simulink model "sst_spdab_npc_inv"  (R2025b)
settings: Solver=ode23tb  StartTime=0.0  StopTime=simlength  FixedStep=tc  MaxStep=tc
values from neighbouring files (symbols this model uses):
  Adrso = eye(2) + Arso*ts_inv    [init_model.m]
  Aresd_max = eye(2) + Ares_max*ts_afe    [init_model.m]
  Aresd_min = eye(2) + Ares_min*ts_afe    [init_model.m]
  Aresd_nom = eye(2) + Ares_nom*ts_afe    [init_model.m]
  Bresd = Bres*ts_afe    [init_model.m]
  CFi_dc2 = 900e-6*4    (= 0.0036)    [init_model.m]
  Cresd = Cres    [init_model.m]
  Crso = [1 0]    [init_model.m]
  delta = 0.025    [init_model.m]
  freq = 50    [init_model.m]
  Iac_FS = I_phase_normalization_factor    [init_model.m]
  Idc_FS = max(Idab1_dc_nom,Idab2_dc_nom) * margin_factor    [init_model.m]
  iph_grid_pu_ref = 3.75    [init_model.m]
  ki_afe = 18    [init_model.m]
  ki_pll = 3140    [init_model.m]
  ki_rpi = 18    [init_model.m]
  kp_afe = 0.25    [init_model.m]
  kp_pll = 314    [init_model.m]
  kp_rpi = 0.25    [init_model.m]
  Ldrso = acker(Adrso',Crso',polesdrso)'    [init_model.m]
  LFu1_AFE = 0.33e-3    (= 0.00033)    [init_model.m]
  n_modules = 2    [init_model.m]
  RLFu1_AFE = 157*0.05*LFu1_AFE    (= 0.0025905)    [init_model.m]
  tc = ts_dab/100    (= 1e-06)    [init_model.m]
  ts_afe = 1/fPWM_AFE    (= 0.0002)    [init_model.m]
  ts_inv = 1/fPWM_INV    (= 0.0002)    [init_model.m]
  Vac_FS = V_phase_normalization_factor    [init_model.m]
  Vdab2_dc_nom = 1500    [init_model.m]
  Vdc_FS = max(Vdab1_dc_nom,Vdab2_dc_nom) * margin_factor    [init_model.m]
undefined symbols (not defined in the file or in its folder): Ld2_trafo, omega_grid_nom, V_phase_normalization_factor
libraries: fl_lib x68, nesl_utility x40, pi_ctrl x4, discrete_time_low_pass_filter x4, dab_single_phase_pwm_modulator x2, full_bridge_mosfet_based_with_thermal_model x2, full_bridge_mosfet_based_with_thermal_model_zvs x2, single_phase_transformer x2, full_bridge_ideal_switch x2, dclink_for_three_levels x2, full_bridge_three_level_npc_ideal_switch_based_model x2, single_phase_three_levels_PWM_modulator x2
(part 3 of 4)

== system sst_spdab_npc_inv/dab_modB/dc//dc with galvanic isolation/full-bridge 1 ==
  gate_commands : Inport
  full-bridge ideal switch based : full_bridge_ideal_switch/full-bridge ideal switch based  Rds_on=Rds_on  Vdon_diode=Vdon_diode  Rdon_diode=Rdon_diode  Csnubber=Csnubber  Rsnubber=Rsnubber  Vth=7.5
  uac_1(+) : PMIOPort  Side=Left
  uac_1(-) : PMIOPort  Port=2  Side=Left
  Udc(+) : PMIOPort  Port=3  Side=Right
  Udc(-) : PMIOPort  Port=4  Side=Right
  wires:
  gate_commands/1 -> full-bridge ideal switch based/1
  connections:
  full-bridge ideal switch based/RConn1 -- uac_1(+)/RConn1
  full-bridge ideal switch based/RConn2 -- uac_1(-)/RConn1
  full-bridge ideal switch based/LConn2 -- Udc(-)/RConn1
  full-bridge ideal switch based/LConn1 -- Udc(+)/RConn1

== system sst_spdab_npc_inv/dab_modB/dc//dc with galvanic isolation/full-bridge 2 ==
  gate_commands : Inport
  CFi_dc2 : fl_lib/Electrical/Electrical Elements/Capacitor  c=CFi_dc2 F  r=RCFi_dc2_internal Ohm  g=0 1/Ohm  i_specify=off  i_priority=None  i=0 A  i_nominal_specify=off  i_nominal_value=1  i_nominal_unit=A  v_specify=off  v_priority=None  v=0 V  v_nominal_specify=off  v_nominal_value=1  v_nominal_unit=V  vc_specify=off  vc_priority=High  vc=0 V  vc_nominal_specify=off  vc_nominal_value=1  vc_nominal_unit=V
  Current Sensor2 : fl_lib/Electrical/Electrical Sensors/Current Sensor
  PS-Simulink Converter6 : nesl_utility/PS-Simulink Converter  PhysicalDomain=network_engine_domain  SubClassName=ps_output  LeftPortType=input  RightPortType=output  PseudoPeriodic=off  Frequencies=[]  VectorFormat=1-D array  Unit=A  AffineConversion=on
  full-bridge ideal switch based : full_bridge_ideal_switch/full-bridge ideal switch based  Rds_on=Rds_on  Vdon_diode=Vdon_diode  Rdon_diode=Rdon_diode  Csnubber=Csnubber  Rsnubber=Rsnubber  Vth=7.5
  uac_1(+) : PMIOPort  Side=Left
  uac_1(-) : PMIOPort  Port=2  Side=Left
  udc(+) : PMIOPort  Port=3  Side=Right
  udc(-) : PMIOPort  Port=4  Side=Right
  tag scope: CFi_dc2_current_modB=global
  wires:
  gate_commands/1 -> full-bridge ideal switch based/1
  PS-Simulink Converter6/1 -> [CFi_dc2_current_modB]  "CFi_dc2_current_modA"
  connections:
  CFi_dc2/LConn1 -- full-bridge ideal switch based/LConn1 -- udc(+)/RConn1
  Current Sensor2/RConn2 -- full-bridge ideal switch based/LConn2 -- udc(-)/RConn1
  PS-Simulink Converter6/LConn1 -- Current Sensor2/RConn1
  CFi_dc2/RConn1 -- Current Sensor2/LConn1
  uac_1(+)/RConn1 -- full-bridge ideal switch based/RConn1
  uac_1(-)/RConn1 -- full-bridge ideal switch based/RConn2

== system sst_spdab_npc_inv/dab_modB/dc//dc with galvanic isolation/scopes ==
  dab TR i2/i1 modB : Scope  NumInputPorts=2
      settings: SampleTime=tc  ActiveDisplayYMinimum=-993.52882611598045  ActiveDisplayYMaximum=1064.2487944856234  DataLoggingVariableName=ScopeData13
  dab TR u2/u1 modB : Scope  NumInputPorts=2
      settings: SampleTime=tc  ActiveDisplayYMinimum=-893.62031856834165  ActiveDisplayYMaximum=653.92363611228757  DataLoggingVariableName=ScopeData4
  dab current output/input modB : Scope  NumInputPorts=2
      settings: SampleTime=tc  ActiveDisplayYMinimum=-7335.7913745283768  ActiveDisplayYMaximum=23819.434208451414  DataLoggingVariableName=ScopeData8
  dab outputs modB : Scope  NumInputPorts=2
      settings: SampleTime=tc  ActiveDisplayYMinimum=-7444.4982322029246  ActiveDisplayYMaximum=21111.562445449617  DataLoggingVariableName=ScopeData6
  dab voltage input/output modB : Scope  NumInputPorts=2
      settings: SampleTime=tc  ActiveDisplayYMinimum=818.889253650666  ActiveDisplayYMaximum=1528.4588304760332  DataLoggingVariableName=ScopeData10
  wires:
  [dab_voltage_input_modB] -> dab voltage input/output modB/1  "dab_voltage_input_modB"
  [dab_current_output_modB] -> dab current output/input modB/1  "dab_current_output_modB"
  [dab_voltage_output_modB] -> dab voltage input/output modB/2  "dab_voltage_output_modB"
  [dab_current_input_modB] -> dab current output/input modB/2  "dab_current_input_modB"
  [i2_dab_transformer_modB] -> dab TR i2/i1 modB/1  "i2_dab_transformer_modB"
  [i1_dab_transformer_modB] -> dab TR i2/i1 modB/2  "i1_dab_transformer_modB"
  [u2_dab_transformer_modB] -> dab TR u2/u1 modB/1  "u2_dab_transformer_modB"
  [u1_dab_transformer_modB] -> dab TR u2/u1 modB/2  "u1_dab_transformer_modB"
  [dab_voltage_output_modB] -> dab outputs modB/2  "dab_voltage_output_modB"
  [dab_current_output_modB] -> dab outputs modB/1  "dab_current_output_modB"

== system sst_spdab_npc_inv/dab_modB/dc//dc with galvanic isolation/single_phase_dab_transformer ==
  Capacitor : fl_lib/Electrical/Electrical Elements/Capacitor  c=Cs1 F  r=1e-6 Ohm  g=0 1/Ohm  i_specify=off  i_priority=None  i=0 A  i_nominal_specify=off  i_nominal_value=1  i_nominal_unit=A  v_specify=off  v_priority=None  v=0 V  v_nominal_specify=off  v_nominal_value=1  v_nominal_unit=V  vc_specify=off  vc_priority=High  vc=0 V  vc_nominal_specify=off  vc_nominal_value=1  vc_nominal_unit=V
  Capacitor1 : fl_lib/Electrical/Electrical Elements/Capacitor  c=Cs2 F  r=1e-6 Ohm  g=0 1/Ohm  i_specify=off  i_priority=None  i=0 A  i_nominal_specify=off  i_nominal_value=1  i_nominal_unit=A  v_specify=off  v_priority=None  v=0 V  v_nominal_specify=off  v_nominal_value=1  v_nominal_unit=V  vc_specify=off  vc_priority=High  vc=0 V  vc_nominal_specify=off  vc_nominal_value=1  vc_nominal_unit=V
  Current Sensor : fl_lib/Electrical/Electrical Sensors/Current Sensor
  Current Sensor1 : fl_lib/Electrical/Electrical Sensors/Current Sensor
  Voltage Sensor1 : fl_lib/Electrical/Electrical Sensors/Voltage Sensor
  Voltage Sensor3 : fl_lib/Electrical/Electrical Sensors/Voltage Sensor
  i1_dab_transformer : nesl_utility/PS-Simulink Converter  PhysicalDomain=network_engine_domain  SubClassName=ps_output  LeftPortType=input  RightPortType=output  PseudoPeriodic=off  Frequencies=[]  VectorFormat=1-D array  Unit=A  AffineConversion=off
  i2_dab_transformer : nesl_utility/PS-Simulink Converter  PhysicalDomain=network_engine_domain  SubClassName=ps_output  LeftPortType=input  RightPortType=output  PseudoPeriodic=off  Frequencies=[]  VectorFormat=1-D array  Unit=A  AffineConversion=off
  single_phase_transformer : single_phase_transformer/single_phase_transformer  lm_trafo=lm_trafo  m1=m1  m2=m2  rd1_trafo=rd1_trafo  rd2_trafo=rd2_trafo  ld1_trafo=ld1_trafo  ld2_trafo=ld2_trafo  rfe_trafo=rfe_trafo  length_core=0.5  mu0=1.256637e-6  mur=70
  single_phase_transformer - scope : Scope
      settings: ActiveDisplayYMinimum=-6.2561553469400835  ActiveDisplayYMaximum=5.3110658573136256  DataLoggingVariableName=ScopeData20
  u1_dab_transformer : nesl_utility/PS-Simulink Converter  PhysicalDomain=network_engine_domain  SubClassName=ps_output  LeftPortType=input  RightPortType=output  PseudoPeriodic=off  Frequencies=[]  VectorFormat=1-D array  Unit=V  AffineConversion=on
  u2_dab_transformer : nesl_utility/PS-Simulink Converter  PhysicalDomain=network_engine_domain  SubClassName=ps_output  LeftPortType=input  RightPortType=output  PseudoPeriodic=off  Frequencies=[]  VectorFormat=1-D array  Unit=V  AffineConversion=on
  u1(+) : PMIOPort  Side=Left
  u2(+) : PMIOPort  Port=2  Side=Right
  u1(-) : PMIOPort  Port=3  Side=Left
  u2(-) : PMIOPort  Port=4  Side=Right
  tag scope: i1_dab_transformer_modB=global, i2_dab_transformer_modB=global, u1_dab_transformer_modB=global, u2_dab_transformer_modB=global
  wires:
  i2_dab_transformer/1 -> [i2_dab_transformer_modB]
  u2_dab_transformer/1 -> [u2_dab_transformer_modB]
  u1_dab_transformer/1 -> [u1_dab_transformer_modB]
  i1_dab_transformer/1 -> [i1_dab_transformer_modB]
  single_phase_transformer/1 -> single_phase_transformer - scope/1
  connections:
  Current Sensor/RConn2 -- u2(+)/RConn1
  Voltage Sensor3/RConn2 -- single_phase_transformer/RConn2 -- u2(-)/RConn1
  Current Sensor/RConn1 -- i2_dab_transformer/LConn1
  Voltage Sensor3/RConn1 -- u2_dab_transformer/LConn1
  Voltage Sensor1/RConn2 -- single_phase_transformer/LConn2 -- u1(-)/RConn1
  Current Sensor1/LConn1 -- Voltage Sensor1/LConn1 -- u1(+)/RConn1
  Voltage Sensor1/RConn1 -- u1_dab_transformer/LConn1
  Current Sensor1/RConn1 -- i1_dab_transformer/LConn1
  Voltage Sensor3/LConn1 -- Capacitor1/RConn1 -- Current Sensor/LConn1
  Capacitor/LConn1 -- Current Sensor1/RConn2
  single_phase_transformer/LConn1 -- Capacitor/RConn1
  single_phase_transformer/RConn1 -- Capacitor1/LConn1

== system sst_spdab_npc_inv/inverter_modA/single phase inverter control1/acquisition_and_scaling_current ==
  in : Inport
  1/Ti5 : Gain  Gain=1/Iac_FS  SaturateOnIntegerOverflow=on  OutDataTypeStr=Inherit: Same as input  ParamDataTypeStr=Inherit: Same as input
  out : Outport
  wires:
  in/1 -> 1/Ti5/1
  1/Ti5/1 -> out/1

== system sst_spdab_npc_inv/inverter_modA/single phase inverter control1/acquisition_and_scaling_dc_voltage ==
  in : Inport
  1/Ti3 : Gain  Gain=1/Vdc_FS  SaturateOnIntegerOverflow=on  OutDataTypeStr=Inherit: Same as input  ParamDataTypeStr=Inherit: Same as input
  out : Outport
  wires:
  in/1 -> 1/Ti3/1
  1/Ti3/1 -> out/1

== system sst_spdab_npc_inv/inverter_modA/single phase inverter control1/acquisition_and_scaling_voltage ==
  in : Inport
  1/Ti5 : Gain  Gain=1/Vac_FS  SaturateOnIntegerOverflow=on  OutDataTypeStr=Inherit: Same as input  ParamDataTypeStr=Inherit: Same as input
  out : Outport
  wires:
  in/1 -> 1/Ti5/1
  1/Ti5/1 -> out/1

== system sst_spdab_npc_inv/inverter_modA/single phase inverter control1/acquisition_and_scaling_voltage1 ==
  in : Inport
  1/Ti1 : Gain  Gain=1/Vac_FS  SaturateOnIntegerOverflow=on  OutDataTypeStr=Inherit: Same as input  ParamDataTypeStr=Inherit: Same as input
  1/Ti2 : Gain  Gain=1/n_modules  SaturateOnIntegerOverflow=on  OutDataTypeStr=Inherit: Same as input  ParamDataTypeStr=Inherit: Same as input
  out : Outport
  wires:
  in/1 -> 1/Ti2/1
  1/Ti1/1 -> out/1
  1/Ti2/1 -> 1/Ti1/1

== system sst_spdab_npc_inv/inverter_modA/single phase inverter control1/inverter_current_output_pu_reference ==
  Gain : Gain  Gain=-1
  Rate Limiter : RateLimiter  RisingSlewLimit=50  FallingSlewLimit=-50  SampleTimeMode=inherited
  Sum : Sum  Inputs=|++
  i_out_inverter_reference_step1 : Step  Time=0.05  After=iph_grid_pu_ref  SampleTime=0
  i_out_inverter_reference_step2 : Step  Commented=on  Time=0.25  After=-iph_grid_pu_ref  SampleTime=0
  inverter_current_output_pu_reference : Outport
  wires:
  Rate Limiter/1 -> Gain/1
  Sum/1 -> Rate Limiter/1
  i_out_inverter_reference_step1/1 -> Sum/1
  i_out_inverter_reference_step2/1 -> Sum/2
  Gain/1 -> inverter_current_output_pu_reference/1

== system sst_spdab_npc_inv/inverter_modA/single phase inverter control1/pwm modulator ==
  vout : Inport
  Constant : Constant  Value=0
  single_phase_three_levels_PWM_generator_with_global_TRGO : single_phase_three_levels_PWM_modulator/single_phase_three_levels_PWM_generator_with_global_TRGO  f=fPWM_INV  m_up=1  m_low=-1  dead_time=dead_time_INV  pos_cmd_gate=15  neg_cmd_gate=-10  polarity=1  tc=tc  double_sampling=TRGO_double_update
  gate_cmds : Outport
  tag scope: TRGO_INV_1=global
  wires:
  vout/1 -> single_phase_three_levels_PWM_generator_with_global_TRGO/3
  [time_afe_module_1] -> single_phase_three_levels_PWM_generator_with_global_TRGO/1
  Constant/1 -> single_phase_three_levels_PWM_generator_with_global_TRGO/2
  single_phase_three_levels_PWM_generator_with_global_TRGO/2 -> gate_cmds/1
  single_phase_three_levels_PWM_generator_with_global_TRGO/1 -> [TRGO_INV_1]

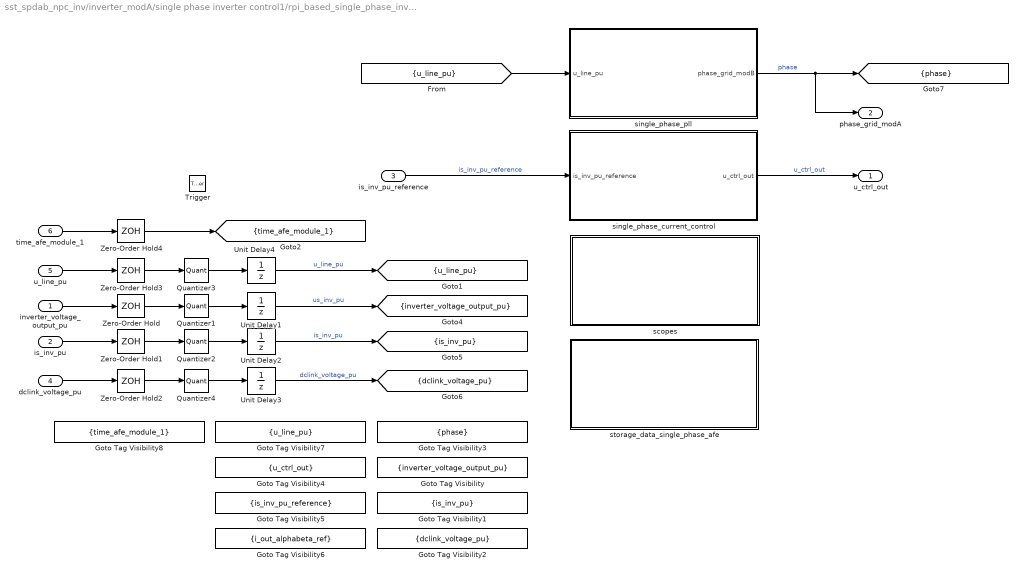
== system sst_spdab_npc_inv/inverter_modA/single phase inverter control1/rpi_based_single_phase_inverter_ctrl ==
  inverter_voltage_output_pu : Inport
  is_inv_pu : Inport  Port=2
  is_inv_pu_reference : Inport  Port=3
  dclink_voltage_pu : Inport  Port=4
  u_line_pu : Inport  Port=5
  time_afe_module_1 : Inport  Port=6
  Trigger : TriggerPort  VariantControl=(inherit)  PortDimensions=1
  Goto Tag Visibility : GotoTagVisibility  GotoTag=inverter_voltage_output_pu
  Goto Tag Visibility1 : GotoTagVisibility  GotoTag=is_inv_pu
  Goto Tag Visibility2 : GotoTagVisibility  GotoTag=dclink_voltage_pu
  Goto Tag Visibility3 : GotoTagVisibility  GotoTag=phase
  Goto Tag Visibility4 : GotoTagVisibility  GotoTag=u_ctrl_out
  Goto Tag Visibility5 : GotoTagVisibility  GotoTag=is_inv_pu_reference
  Goto Tag Visibility6 : GotoTagVisibility  GotoTag=i_out_alphabeta_ref
  Goto Tag Visibility7 : GotoTagVisibility  GotoTag=u_line_pu
  Goto Tag Visibility8 : GotoTagVisibility  GotoTag=time_afe_module_1
  Quantizer{1..4} (4 alike) : Quantizer  QuantizationInterval=adc12_quantization
  Unit Delay{1..4} (4 alike) : UnitDelay  SampleTime=-1  HasFrameUpgradeWarning=on
  Zero-Order Hold{,1..4} (5 alike) : ZeroOrderHold  SampleTime=-1
  scopes : Subsystem
  single_phase_current_control : Subsystem
  single_phase_pll : Subsystem
  storage_data_single_phase_afe : Subsystem
  u_ctrl_out : Outport
  phase_grid_modA : Outport  Port=2
  tag scope: dclink_voltage_pu=scoped, inverter_voltage_output_pu=scoped, is_inv_pu=scoped, phase=scoped, time_afe_module_1=scoped, u_line_pu=scoped
  wires:
  inverter_voltage_output_pu/1 -> Zero-Order Hold/1
  is_inv_pu/1 -> Zero-Order Hold1/1
  dclink_voltage_pu/1 -> Zero-Order Hold2/1
  Unit Delay1/1 -> [inverter_voltage_output_pu]  "us_inv_pu"
  Unit Delay2/1 -> [is_inv_pu]  "is_inv_pu"
  Unit Delay3/1 -> [dclink_voltage_pu]  "dclink_voltage_pu"
  is_inv_pu_reference/1 -> single_phase_current_control/1(is_inv_pu_reference)  "is_inv_pu_reference"
  single_phase_current_control/1(u_ctrl_out) -> u_ctrl_out/1  "u_ctrl_out"
  u_line_pu/1 -> Zero-Order Hold3/1
  Quantizer1/1 -> Unit Delay1/1
  Quantizer2/1 -> Unit Delay2/1
  Quantizer4/1 -> Unit Delay3/1
  Quantizer3/1 -> Unit Delay4/1
  single_phase_pll/1(phase_grid_modB) -> phase_grid_modA/1, [phase]  "phase"
  Zero-Order Hold/1 -> Quantizer1/1
  Zero-Order Hold1/1 -> Quantizer2/1
  Zero-Order Hold2/1 -> Quantizer4/1
  Unit Delay4/1 -> [u_line_pu]  "u_line_pu"
  [u_line_pu] -> single_phase_pll/1(u_line_pu)
  Zero-Order Hold3/1 -> Quantizer3/1
  time_afe_module_1/1 -> Zero-Order Hold4/1
  Zero-Order Hold4/1 -> [time_afe_module_1]

== system sst_spdab_npc_inv/inverter_modB/single phase inverter control1/acquisition_and_scaling_current ==
  in : Inport
  1/Ti5 : Gain  Gain=1/Iac_FS  SaturateOnIntegerOverflow=on  OutDataTypeStr=Inherit: Same as input  ParamDataTypeStr=Inherit: Same as input
  out : Outport
  wires:
  in/1 -> 1/Ti5/1
  1/Ti5/1 -> out/1

== system sst_spdab_npc_inv/inverter_modB/single phase inverter control1/acquisition_and_scaling_dc_voltage ==
  in : Inport
  1/Ti3 : Gain  Gain=1/Vdc_FS  SaturateOnIntegerOverflow=on  OutDataTypeStr=Inherit: Same as input  ParamDataTypeStr=Inherit: Same as input
  out : Outport
  wires:
  in/1 -> 1/Ti3/1
  1/Ti3/1 -> out/1

== system sst_spdab_npc_inv/inverter_modB/single phase inverter control1/acquisition_and_scaling_voltage ==
  in : Inport
  1/Ti5 : Gain  Gain=1/Vac_FS  SaturateOnIntegerOverflow=on  OutDataTypeStr=Inherit: Same as input  ParamDataTypeStr=Inherit: Same as input
  out : Outport
  wires:
  in/1 -> 1/Ti5/1
  1/Ti5/1 -> out/1

== system sst_spdab_npc_inv/inverter_modB/single phase inverter control1/acquisition_and_scaling_voltage1 ==
  in : Inport
  1/Ti1 : Gain  Gain=1/Vac_FS  SaturateOnIntegerOverflow=on  OutDataTypeStr=Inherit: Same as input  ParamDataTypeStr=Inherit: Same as input
  1/Ti2 : Gain  Gain=1/n_modules  SaturateOnIntegerOverflow=on  OutDataTypeStr=Inherit: Same as input  ParamDataTypeStr=Inherit: Same as input
  out : Outport
  wires:
  in/1 -> 1/Ti2/1
  1/Ti1/1 -> out/1
  1/Ti2/1 -> 1/Ti1/1

== system sst_spdab_npc_inv/inverter_modB/single phase inverter control1/inverter_current_output_pu_reference ==
  Gain : Gain
  Rate Limiter : RateLimiter  RisingSlewLimit=50  FallingSlewLimit=-50  SampleTimeMode=inherited
  Sum : Sum  Inputs=|++
  i_out_inverter_reference_step1 : Step  Time=0.05  After=iph_grid_pu_ref  SampleTime=0
  i_out_inverter_reference_step2 : Step  Commented=on  Time=0.25  After=-iph_grid_pu_ref  SampleTime=0
  inverter_current_output_pu_reference : Outport
  wires:
  Rate Limiter/1 -> Gain/1
  Sum/1 -> Rate Limiter/1
  i_out_inverter_reference_step1/1 -> Sum/1
  i_out_inverter_reference_step2/1 -> Sum/2
  Gain/1 -> inverter_current_output_pu_reference/1

== system sst_spdab_npc_inv/inverter_modB/single phase inverter control1/pwm modulator ==
  vout : Inport
  Constant : Constant  Value=0
  single_phase_three_levels_PWM_generator_with_global_TRGO : single_phase_three_levels_PWM_modulator/single_phase_three_levels_PWM_generator_with_global_TRGO  f=fPWM_INV  m_up=1  m_low=-1  dead_time=dead_time_INV  pos_cmd_gate=15  neg_cmd_gate=-10  polarity=1  tc=tc  double_sampling=TRGO_double_update
  gate_cmds : Outport
  tag scope: TRGO_INV_2=global
  wires:
  vout/1 -> single_phase_three_levels_PWM_generator_with_global_TRGO/3
  Constant/1 -> single_phase_three_levels_PWM_generator_with_global_TRGO/2
  single_phase_three_levels_PWM_generator_with_global_TRGO/2 -> gate_cmds/1
  single_phase_three_levels_PWM_generator_with_global_TRGO/1 -> [TRGO_INV_2]
  [time_afe_module_2] -> single_phase_three_levels_PWM_generator_with_global_TRGO/1

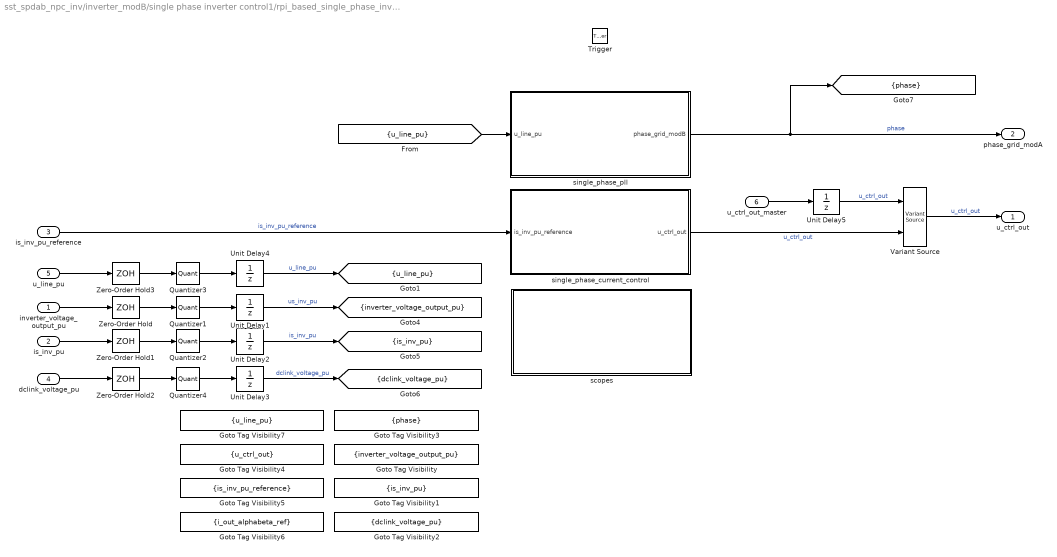
== system sst_spdab_npc_inv/inverter_modB/single phase inverter control1/rpi_based_single_phase_inverter_ctrl ==
  inverter_voltage_output_pu : Inport
  is_inv_pu : Inport  Port=2
  is_inv_pu_reference : Inport  Port=3
  dclink_voltage_pu : Inport  Port=4
  u_line_pu : Inport  Port=5
  u_ctrl_out_master : Inport  Port=6
  Trigger : TriggerPort  VariantControl=(inherit)  PortDimensions=1
  Goto Tag Visibility : GotoTagVisibility  GotoTag=inverter_voltage_output_pu
  Goto Tag Visibility1 : GotoTagVisibility  GotoTag=is_inv_pu
  Goto Tag Visibility2 : GotoTagVisibility  GotoTag=dclink_voltage_pu
  Goto Tag Visibility3 : GotoTagVisibility  GotoTag=phase
  Goto Tag Visibility4 : GotoTagVisibility  GotoTag=u_ctrl_out
  Goto Tag Visibility5 : GotoTagVisibility  GotoTag=is_inv_pu_reference
  Goto Tag Visibility6 : GotoTagVisibility  GotoTag=i_out_alphabeta_ref
  Goto Tag Visibility7 : GotoTagVisibility  GotoTag=u_line_pu
  Quantizer{1..4} (4 alike) : Quantizer  QuantizationInterval=adc12_quantization
  Unit Delay{1..5} (5 alike) : UnitDelay  SampleTime=-1  HasFrameUpgradeWarning=on
  Variant Source : VariantSource  VariantControls={true, false}
  Zero-Order Hold{,1..3} (4 alike) : ZeroOrderHold  SampleTime=-1
  scopes : Subsystem
  single_phase_current_control : Subsystem
  single_phase_pll : Subsystem
  u_ctrl_out : Outport
  phase_grid_modA : Outport  Port=2
  tag scope: dclink_voltage_pu=scoped, inverter_voltage_output_pu=scoped, is_inv_pu=scoped, phase=scoped, u_line_pu=scoped
  wires:
  inverter_voltage_output_pu/1 -> Zero-Order Hold/1
  is_inv_pu/1 -> Zero-Order Hold1/1
  dclink_voltage_pu/1 -> Zero-Order Hold2/1
  Unit Delay1/1 -> [inverter_voltage_output_pu]  "us_inv_pu"
  Unit Delay2/1 -> [is_inv_pu]  "is_inv_pu"
  Unit Delay3/1 -> [dclink_voltage_pu]  "dclink_voltage_pu"
  is_inv_pu_reference/1 -> single_phase_current_control/1(is_inv_pu_reference)  "is_inv_pu_reference"
  u_line_pu/1 -> Zero-Order Hold3/1
  Quantizer1/1 -> Unit Delay1/1
  Quantizer2/1 -> Unit Delay2/1
  Quantizer4/1 -> Unit Delay3/1
  Quantizer3/1 -> Unit Delay4/1
  single_phase_pll/1(phase_grid_modB) -> [phase], phase_grid_modA/1  "phase"
  Zero-Order Hold/1 -> Quantizer1/1
  Zero-Order Hold1/1 -> Quantizer2/1
  Zero-Order Hold2/1 -> Quantizer4/1
  Unit Delay4/1 -> [u_line_pu]  "u_line_pu"
  [u_line_pu] -> single_phase_pll/1(u_line_pu)
  Zero-Order Hold3/1 -> Quantizer3/1
  u_ctrl_out_master/1 -> Unit Delay5/1
  Unit Delay5/1 -> Variant Source/1  "u_ctrl_out"
  Variant Source/1 -> u_ctrl_out/1  "u_ctrl_out"
  single_phase_current_control/1(u_ctrl_out) -> Variant Source/2  "u_ctrl_out"

== system sst_spdab_npc_inv/dab_modA/dab_ctrl/dab_voltage&current_controllers/input current controller ==
  i_in_dab_ref : Inport
  i_in_dab : Inport  Port=2
  Gain : Gain
  dab_current_control performance_modA : Scope  NumInputPorts=3
      settings: ActiveDisplayYMinimum=-1.3198512407012277  ActiveDisplayYMaximum=3.2550260581251234  DataLoggingVariableName=ScopeData12
  pi_ctrl : pi_ctrl/pi_ctrl  kp=kp_i_dab  ki=ki_i_dab  ts=ts_dab  lim_up=1  lim_down=-1
  i_ctrl_out : Outport
  wires:
  i_in_dab_ref/1 -> pi_ctrl/1, dab_current_control performance_modA/1, Gain/1  "i_in_dab_ref"
  i_in_dab/1 -> pi_ctrl/2, dab_current_control performance_modA/2  "i_in_dab"
  pi_ctrl/1 -> i_ctrl_out/1, dab_current_control performance_modA/3  "i_ctrl_out"
  Gain/1 -> pi_ctrl/3

== system sst_spdab_npc_inv/dab_modA/dab_ctrl/dab_voltage&current_controllers/output voltage controller ==
  u_out_dab_ref : Inport
  u_out_dab : Inport  Port=2
  dab_voltage_control performance_modA : Scope  NumInputPorts=3
      settings: ActiveDisplayYMinimum=-1.3198512407012277  ActiveDisplayYMaximum=3.2550260581251234  DataLoggingVariableName=ScopeData14
  pi_ctrl : pi_ctrl/pi_ctrl  kp=kp_v_dab  ki=ki_v_dab  ts=ts_dab  lim_up=4  lim_down=-4
  u_ctrl_out : Outport
  wires:
  u_out_dab/1 -> dab_voltage_control performance_modA/2, pi_ctrl/2  "u_out_dab"
  u_out_dab_ref/1 -> dab_voltage_control performance_modA/1, pi_ctrl/1  "u_out_dab_ref"
  pi_ctrl/1 -> dab_voltage_control performance_modA/3, u_ctrl_out/1  "u_ctrl_out"

== system sst_spdab_npc_inv/dab_modA/dab_ctrl/dab_voltage&current_controllers/scopes ==
  Bus Creator : BusCreator  Inputs=2
  Bus Creator1 : BusCreator  Inputs=2
  dab-tracking modA : Scope  NumInputPorts=2
      settings: ActiveDisplayYMinimum=-2.2033655574404327  ActiveDisplayYMaximum=2.9011172646804795  DataLoggingVariableName=ScopeData7
  u_ctrl_out_dab/i_ctrl_out_dab modA : Scope  NumInputPorts=2
      settings: ActiveDisplayYMinimum=-1.25  ActiveDisplayYMaximum=1.25
  wires:
  [dab_current_input_pu] -> Bus Creator1/2  "dab_current_input_pu"
  [dab_current_ctrl_output_pu] -> u_ctrl_out_dab/i_ctrl_out_dab modA/2  "i_ctrl_out_dab"
  [dab_voltage_output_pu] -> Bus Creator/2  "dab_voltage_output_pu"
  [dab_voltage_output_pu_reference] -> Bus Creator/1  "dab_current_input_pu_ref"
  Bus Creator1/1 -> dab-tracking modA/2
  Bus Creator/1 -> dab-tracking modA/1
  [dab_voltage_ctrl_output_pu] -> u_ctrl_out_dab/i_ctrl_out_dab modA/1  "u_ctrl_out_dab"
  [dab_voltage_ctrl_output_pu] -> Bus Creator1/1  "u_ctrl_out_dab"

== system sst_spdab_npc_inv/dab_modA/dab_ctrl/dab_voltage&current_controllers/storage_data_dab ==
  To Workspace1 : ToWorkspace  VariableName=time_ts_dab_sim  SampleTime=-1
      settings: MaxDataPoints=Ns_dab
  To Workspace2 : ToWorkspace  VariableName=dab_current_input_pu_ref_sim  SampleTime=-1
      settings: MaxDataPoints=Ns_dab
  To Workspace3 : ToWorkspace  VariableName=dab_voltage_output_pu_sim  SampleTime=-1
      settings: MaxDataPoints=Ns_dab
  To Workspace5 : ToWorkspace  VariableName=dab_current_input_pu_sim  SampleTime=-1
      settings: MaxDataPoints=Ns_dab
  To Workspace6 : ToWorkspace  VariableName=u_ctrl_out_dab_sim  SampleTime=-1
      settings: MaxDataPoints=Ns_dab
  To Workspace7 : ToWorkspace  VariableName=i_ctrl_out_dab_sim  SampleTime=-1
      settings: MaxDataPoints=Ns_dab
  wires:
  [dab_voltage_ctrl_output_pu] -> To Workspace6/1  "u_ctrl_out_dab"
  [dab_voltage_output_pu_reference] -> To Workspace2/1  "dab_current_input_pu_ref"
  [dab_voltage_output_pu] -> To Workspace3/1  "dab_voltage_output_pu"
  [dab_current_ctrl_output_pu] -> To Workspace7/1  "i_ctrl_out_dab"
  [dab_current_input_pu] -> To Workspace5/1  "dab_current_input_pu"
  [time_dab_module_1] -> To Workspace1/1

== system sst_spdab_npc_inv/dab_modB/dab_ctrl/dab_voltage&current_controllers/input current controller ==
  i_in_dab_ref : Inport
  i_in_dab : Inport  Port=2
  Gain : Gain
  dab_current_control performance_modB : Scope  NumInputPorts=3
      settings: ActiveDisplayYMinimum=-1.3198512407012277  ActiveDisplayYMaximum=3.2550260581251234  DataLoggingVariableName=ScopeData12
  pi_ctrl : pi_ctrl/pi_ctrl  kp=kp_i_dab  ki=ki_i_dab  ts=ts_dab  lim_up=1  lim_down=-1
  i_ctrl_out : Outport
  wires:
  i_in_dab_ref/1 -> pi_ctrl/1, dab_current_control performance_modB/1, Gain/1  "i_in_dab_ref"
  i_in_dab/1 -> pi_ctrl/2, dab_current_control performance_modB/2  "i_in_dab"
  pi_ctrl/1 -> i_ctrl_out/1, dab_current_control performance_modB/3  "i_ctrl_out"
  Gain/1 -> pi_ctrl/3

== system sst_spdab_npc_inv/dab_modB/dab_ctrl/dab_voltage&current_controllers/output voltage controller ==
  u_out_dab_ref : Inport
  u_out_dab : Inport  Port=2
  dab_voltage_control performance_modB : Scope  NumInputPorts=3
      settings: ActiveDisplayYMinimum=-0.72078430609168342  ActiveDisplayYMaximum=1.2253779437324093  DataLoggingVariableName=ScopeData14
  pi_ctrl : pi_ctrl/pi_ctrl  kp=kp_v_dab  ki=ki_v_dab  ts=ts_dab  lim_up=4  lim_down=-4
  u_ctrl_out : Outport
  wires:
  u_out_dab/1 -> dab_voltage_control performance_modB/2, pi_ctrl/2  "u_out_dab"
  u_out_dab_ref/1 -> dab_voltage_control performance_modB/1, pi_ctrl/1  "u_out_dab_ref"
  pi_ctrl/1 -> dab_voltage_control performance_modB/3, u_ctrl_out/1  "u_ctrl_out"

== system sst_spdab_npc_inv/dab_modB/dab_ctrl/dab_voltage&current_controllers/scopes ==
  Bus Creator : BusCreator  Inputs=2
  Bus Creator1 : BusCreator  Inputs=2
  dab-tracking modB : Scope  NumInputPorts=2
      settings: ActiveDisplayYMinimum=-2.2033655574404327  ActiveDisplayYMaximum=2.9011172646804795  DataLoggingVariableName=ScopeData7
  u_ctrl_out_dab/i_ctrl_out_dab modB : Scope  NumInputPorts=2
      settings: ActiveDisplayYMinimum=-1.25  ActiveDisplayYMaximum=1.25
  wires:
  [dab_current_input_pu] -> Bus Creator1/2  "dab_current_input_pu"
  [dab_current_ctrl_output_pu] -> u_ctrl_out_dab/i_ctrl_out_dab modB/2  "i_ctrl_out_dab"
  [dab_voltage_output_pu] -> Bus Creator/2  "dab_voltage_output_pu"
  [dab_voltage_output_pu_reference] -> Bus Creator/1  "dab_current_input_pu_ref"
  Bus Creator1/1 -> dab-tracking modB/2
  Bus Creator/1 -> dab-tracking modB/1
  [dab_voltage_ctrl_output_pu] -> u_ctrl_out_dab/i_ctrl_out_dab modB/1  "u_ctrl_out_dab"
  [dab_voltage_ctrl_output_pu] -> Bus Creator1/1  "u_ctrl_out_dab"

== system sst_spdab_npc_inv/inverter_modA/single phase inverter control1/rpi_based_single_phase_inverter_ctrl/scopes ==
  Bus Creator1 : BusCreator  Inputs=3
  Bus Creator2 : BusCreator  Inputs=2
  Bus Creator3 : BusCreator  Inputs=2
  Bus Creator4 : BusCreator  Inputs=2
  single phase inverter tracking current scope 1 : Scope  NumInputPorts=2
      settings: ActiveDisplayYMinimum=-3.13873291015625  ActiveDisplayYMaximum=3.12652587890625  DataLoggingVariableName=ScopeData12
  single phase inverter tracking current scope 2 : Scope  NumInputPorts=2
      settings: ActiveDisplayYMinimum=-9.9064807170854827  ActiveDisplayYMaximum=9.6151714521585063  DataLoggingVariableName=ScopeData2
  single phase inverter tracking current scope 3 : Scope  NumInputPorts=2
      settings: ActiveDisplayYMinimum=-9.9064807170854827  ActiveDisplayYMaximum=9.6151714521585063  DataLoggingVariableName=ScopeData21
  wires:
  Bus Creator1/1 -> single phase inverter tracking current scope 1/2  "is_tracking"
  [i_out_alphabeta_ref] -> Bus Creator1/2  "i_out_inverter_pu_ref"
  [is_inv_pu] -> Bus Creator1/3  "inverter_current_output_pu"
  [inverter_voltage_output_pu] -> Bus Creator2/1  "inverter_voltage_output_pu"
  Bus Creator2/1 -> single phase inverter tracking current scope 1/1  "load"
  [is_inv_pu_reference] -> Bus Creator1/1  "inverter_current_output_pu_reference"
  [is_inv_pu] -> Bus Creator2/2  "inverter_current_output_pu"
  [u_ctrl_out] -> Bus Creator3/1  "u_ctrl_out"
  [inverter_voltage_output_pu] -> Bus Creator3/2  "inverter_voltage_output_pu"
  Bus Creator3/1 -> single phase inverter tracking current scope 2/2  "u_load"
  [is_inv_pu] -> Bus Creator4/2  "inverter_current_output_pu"
  [i_out_alphabeta_ref] -> Bus Creator4/1  "i_out_alphabeta_ref"
  Bus Creator4/1 -> single phase inverter tracking current scope 2/1  "i_load"
  [phase] -> single phase inverter tracking current scope 3/1  "phase_pll"

== system sst_spdab_npc_inv/inverter_modA/single phase inverter control1/rpi_based_single_phase_inverter_ctrl/single_phase_current_control ==
  is_inv_pu_reference : Inport
  Variant Source : VariantSource  VariantControls={rpi_enable == 1, rpi_enable == 0}
  current_reference_generation : Subsystem
  dqpi_current_controller : Subsystem
  rpi_current_controller : Subsystem
  u_ctrl_out : Outport
  tag scope: i_out_alphabeta_ref=scoped, is_inv_pu_reference=scoped, u_ctrl_out=scoped
  wires:
  rpi_current_controller/1(u_ctrl_out) -> Variant Source/1  "u_ctrl_out"
  dqpi_current_controller/1(u_out) -> Variant Source/2  "u_ctrl_out"
  current_reference_generation/1(is_ref) -> rpi_current_controller/1(i_ref), [i_out_alphabeta_ref]  "i_out_inverter_pu_ref"
  Variant Source/1 -> u_ctrl_out/1, [u_ctrl_out]  "u_ctrl_out"
  [phase] -> current_reference_generation/2(phase)
  is_inv_pu_reference/1 -> current_reference_generation/1(mag_ref), [is_inv_pu_reference]
  current_reference_generation/2(idc_ref) -> dqpi_current_controller/1(i_ref)

== system sst_spdab_npc_inv/inverter_modA/single phase inverter control1/rpi_based_single_phase_inverter_ctrl/single_phase_pll ==
  u_line_pu : Inport
  Constant : Constant  Value=2*pi*freq
  Constant2 : Constant  Value=0
  Sum : Sum  Inputs=|++
  Sum1 : Sum  Inputs=|++
  Terminator1 : Terminator
  Terminator2 : Terminator
  Terminator3 : Terminator
  Unit Delay1 : UnitDelay  SampleTime=-1  HasFrameUpgradeWarning=on
  alphabeta2xieta : MATLAB Function  TreatAsAtomicUnit=on
  double_integrator_observer : Subsystem
  freq_pll : Gain  Gain=1/2/pi
  omega_int_ts : Gain  Gain=ts_inv
  pi-ctrl : Subsystem  mask{kp=kp_pll, ki=ki_pll, ts=ts_afe, sat_pos=inf, sat_neg=-inf}
  theta_pll_hat : Gain
  ualpha_pll : Gain
  ubeta_pll : Gain
  ueta_pll : Gain  Gain=-1
  ueta_pll_flt : discrete_time_low_pass_filter/discrete-time-low-pass-filter  tau=tau_f  ts=ts_afe
  uxi_pll : Gain
  uxi_pll_flt : discrete_time_low_pass_filter/discrete-time-low-pass-filter  tau=tau_f  ts=ts_afe
  xieta2alphabeta : MATLAB Function  TreatAsAtomicUnit=on
  phase_grid_modB : Outport
  wires:
  Sum/1 -> Unit Delay1/1
  alphabeta2xieta/1(xi) -> uxi_pll_flt/1, uxi_pll/1
  xieta2alphabeta/2(beta) -> ubeta_pll/1
  alphabeta2xieta/2(eta) -> ueta_pll_flt/1, ueta_pll/1
  omega_int_ts/1 -> Sum/1
  double_integrator_observer/1(theta_hat) -> theta_pll_hat/1  "theta_hat"
  u_line_pu/1 -> alphabeta2xieta/1(alpha)
  freq_pll/1 -> Terminator1/1  "freq_pll"
  ueta_pll_flt/1 -> xieta2alphabeta/2(eta)
  uxi_pll_flt/1 -> xieta2alphabeta/1(xi)
  ueta_pll/1 -> pi-ctrl/1(x)
  Sum1/1 -> freq_pll/1, omega_int_ts/1  "freq_pll"
  Constant2/1 -> pi-ctrl/2(xref)
  uxi_pll/1 -> Terminator2/1
  ubeta_pll/1 -> alphabeta2xieta/2(beta)
  xieta2alphabeta/1(alpha) -> ualpha_pll/1
  ualpha_pll/1 -> Terminator3/1
  pi-ctrl/1(u) -> Sum1/1
  Constant/1 -> Sum1/2
  theta_pll_hat/1 -> phase_grid_modB/1  "theta_pll_hat"
  Unit Delay1/1 -> Sum/2, double_integrator_observer/1(theta), xieta2alphabeta/3(gamma), alphabeta2xieta/3(gamma)

== system sst_spdab_npc_inv/inverter_modA/single phase inverter control1/rpi_based_single_phase_inverter_ctrl/storage_data_single_phase_afe ==
  Bus Selector : BusSelector  OutputSignals=is_ref_alpha
  To Workspace1 : ToWorkspace  VariableName=time_ts_afe_sim  SampleTime=-1
      settings: MaxDataPoints=Ns_afe
  To Workspace2 : ToWorkspace  VariableName=is_inv_pu_reference_sim  SampleTime=-1
      settings: MaxDataPoints=Ns_afe
  To Workspace3 : ToWorkspace  VariableName=is_inv_pu_sim  SampleTime=-1
      settings: MaxDataPoints=Ns_afe
  To Workspace4 : ToWorkspace  VariableName=is_ref_alpha_sim  SampleTime=-1
      settings: MaxDataPoints=Ns_afe
  To Workspace5 : ToWorkspace  VariableName=u_ctrl_out_sim  SampleTime=-1
      settings: MaxDataPoints=Ns_afe
  wires:
  [is_inv_pu_reference] -> To Workspace2/1  "is_inv_pu_reference"
  [is_inv_pu] -> To Workspace3/1  "is_inv_pu"
  [i_out_alphabeta_ref] -> Bus Selector/1  "i_out_inverter_pu_ref"
  Bus Selector/1 -> To Workspace4/1  "<is_ref_alpha>"
  [u_ctrl_out] -> To Workspace5/1  "u_ctrl_out"
  [time_afe_module_1] -> To Workspace1/1

== system sst_spdab_npc_inv/inverter_modB/single phase inverter control1/rpi_based_single_phase_inverter_ctrl/scopes ==
  Bus Creator1 : BusCreator  Inputs=3
  Bus Creator2 : BusCreator  Inputs=2
  Bus Creator3 : BusCreator  Inputs=2
  Bus Creator4 : BusCreator  Inputs=2
  single phase inverter tracking current scope 1 : Scope  NumInputPorts=2
      settings: ActiveDisplayYMinimum=-3.13873291015625  ActiveDisplayYMaximum=3.12652587890625  DataLoggingVariableName=ScopeData12
  single phase inverter tracking current scope 2 : Scope  NumInputPorts=2
      settings: ActiveDisplayYMinimum=-5.08172607421875  ActiveDisplayYMaximum=4.05096435546875  DataLoggingVariableName=ScopeData2
  wires:
  Bus Creator1/1 -> single phase inverter tracking current scope 1/2  "is_tracking"
  [i_out_alphabeta_ref] -> Bus Creator1/2  "i_out_inverter_pu_ref"
  [is_inv_pu] -> Bus Creator1/3  "inverter_current_output_pu"
  [inverter_voltage_output_pu] -> Bus Creator2/1  "inverter_voltage_output_pu"
  Bus Creator2/1 -> single phase inverter tracking current scope 1/1  "load"
  [is_inv_pu_reference] -> Bus Creator1/1  "inverter_current_output_pu_reference"
  [is_inv_pu] -> Bus Creator2/2  "inverter_current_output_pu"
  [u_ctrl_out] -> Bus Creator3/1  "u_ctrl_out"
  [inverter_voltage_output_pu] -> Bus Creator3/2  "inverter_voltage_output_pu"
  Bus Creator3/1 -> single phase inverter tracking current scope 2/2  "u_load"
  [is_inv_pu] -> Bus Creator4/2  "inverter_current_output_pu"
  [i_out_alphabeta_ref] -> Bus Creator4/1  "i_out_alphabeta_ref"
  Bus Creator4/1 -> single phase inverter tracking current scope 2/1  "i_load"

== system sst_spdab_npc_inv/inverter_modB/single phase inverter control1/rpi_based_single_phase_inverter_ctrl/single_phase_current_control ==
  is_inv_pu_reference : Inport
  Variant Source : VariantSource  VariantControls={rpi_enable == 1, rpi_enable == 0}
  current_reference_generation : Subsystem
  dqpi_current_controller : Subsystem
  rpi_current_controller : Subsystem
  u_ctrl_out : Outport
  tag scope: i_out_alphabeta_ref=scoped, is_inv_pu_reference=scoped, u_ctrl_out=scoped
  wires:
  rpi_current_controller/1(u_ctrl_out) -> Variant Source/1  "u_ctrl_out"
  dqpi_current_controller/1(u_out) -> Variant Source/2  "u_ctrl_out"
  current_reference_generation/1(is_ref) -> rpi_current_controller/1(i_ref), [i_out_alphabeta_ref]  "i_out_inverter_pu_ref"
  Variant Source/1 -> u_ctrl_out/1, [u_ctrl_out]  "u_ctrl_out"
  [phase] -> current_reference_generation/2(phase)
  is_inv_pu_reference/1 -> current_reference_generation/1(mag_ref), [is_inv_pu_reference]
  current_reference_generation/2(idc_ref) -> dqpi_current_controller/1(i_ref)

== system sst_spdab_npc_inv/inverter_modB/single phase inverter control1/rpi_based_single_phase_inverter_ctrl/single_phase_pll ==
  u_line_pu : Inport
  Constant : Constant  Value=2*pi*freq
  Constant2 : Constant  Value=0
  Sum : Sum  Inputs=|++
  Sum1 : Sum  Inputs=|++
  Terminator1 : Terminator
  Terminator2 : Terminator
  Terminator3 : Terminator
  Unit Delay1 : UnitDelay  SampleTime=-1  HasFrameUpgradeWarning=on
  alphabeta2xieta : MATLAB Function  TreatAsAtomicUnit=on
  double_integrator_observer : Subsystem
  freq_pll : Gain  Gain=1/2/pi
  omega_int_ts : Gain  Gain=ts_inv
  pi-ctrl : Subsystem  mask{kp=kp_pll, ki=ki_pll, ts=ts_afe, sat_pos=inf, sat_neg=-inf}
  theta_pll_hat : Gain
  ualpha_pll : Gain
  ubeta_pll : Gain
  ueta_pll : Gain  Gain=-1
  ueta_pll_flt : discrete_time_low_pass_filter/discrete-time-low-pass-filter  tau=tau_f  ts=ts_afe
  uxi_pll : Gain
  uxi_pll_flt : discrete_time_low_pass_filter/discrete-time-low-pass-filter  tau=tau_f  ts=ts_afe
  xieta2alphabeta : MATLAB Function  TreatAsAtomicUnit=on
  phase_grid_modB : Outport
  wires:
  Sum/1 -> Unit Delay1/1
  alphabeta2xieta/1(xi) -> uxi_pll_flt/1, uxi_pll/1
  xieta2alphabeta/2(beta) -> ubeta_pll/1
  alphabeta2xieta/2(eta) -> ueta_pll_flt/1, ueta_pll/1
  omega_int_ts/1 -> Sum/1
  double_integrator_observer/1(theta_hat) -> theta_pll_hat/1  "theta_hat"
  u_line_pu/1 -> alphabeta2xieta/1(alpha)
  freq_pll/1 -> Terminator1/1  "freq_pll"
  ueta_pll_flt/1 -> xieta2alphabeta/2(eta)
  uxi_pll_flt/1 -> xieta2alphabeta/1(xi)
  ueta_pll/1 -> pi-ctrl/1(x)
  Sum1/1 -> freq_pll/1, omega_int_ts/1  "freq_pll"
  Constant2/1 -> pi-ctrl/2(xref)
  uxi_pll/1 -> Terminator2/1
  ubeta_pll/1 -> alphabeta2xieta/2(beta)
  xieta2alphabeta/1(alpha) -> ualpha_pll/1
  ualpha_pll/1 -> Terminator3/1
  pi-ctrl/1(u) -> Sum1/1
  Constant/1 -> Sum1/2
  theta_pll_hat/1 -> phase_grid_modB/1  "theta_pll_hat"
  Unit Delay1/1 -> Sum/2, double_integrator_observer/1(theta), xieta2alphabeta/3(gamma), alphabeta2xieta/3(gamma)

== system sst_spdab_npc_inv/inverter_modA/single phase inverter control1/rpi_based_single_phase_inverter_ctrl/single_phase_current_control/current_reference_generation ==
  mag_ref : Inport
  phase : Inport  Port=2
  Bus Creator : BusCreator  Inputs=2
  Product : Product
  Product1 : Product
  Sin : Trigonometry  Operator=cos
  Sin1 : Trigonometry
  is_ref : Outport
  idc_ref : Outport  Port=2
  wires:
  Sin/1 -> Product/2
  phase/1 -> Sin1/1, Sin/1
  mag_ref/1 -> idc_ref/1, Product1/1, Product/1
  Sin1/1 -> Product1/2
  Product/1 -> Bus Creator/1  "is_ref_alpha"
  Product1/1 -> Bus Creator/2  "is_ref_beta"
  Bus Creator/1 -> is_ref/1

== system sst_spdab_npc_inv/inverter_modA/single phase inverter control1/rpi_based_single_phase_inverter_ctrl/single_phase_current_control/dqpi_current_controller ==
  i_ref : Inport
  alphabeta2dq : Subsystem
  dq2alphabeta : Subsystem
  dq_vector_pi : Subsystem
  i_alpha_beta : Scope  NumInputPorts=2
      settings: ActiveDisplayYMinimum=-5.6739147526013909  ActiveDisplayYMaximum=4.7712874609125189  DataLoggingVariableName=ScopeData2
  phase shift filter1 : phase_shift_filter/phase shift filter  f=omega_grid_nom/2/pi  ts=ts_afe
  u_out : Outport
  wires:
  dq2alphabeta/1(alpha) -> u_out/1
  [is_inv_pu] -> phase shift filter1/1, i_alpha_beta/1, alphabeta2dq/1(alpha)  "i_alpha"
  phase shift filter1/1 -> i_alpha_beta/2, alphabeta2dq/2(beta)  "i_beta"
  i_ref/1 -> dq_vector_pi/1(id_ref)  "id_ref"
  alphabeta2dq/1("d ") -> dq_vector_pi/2(id)  "id"
  alphabeta2dq/2("q ") -> dq_vector_pi/3(iq)  "iq"
  dq_vector_pi/1(ud_ctrl) -> dq2alphabeta/1(d)
  dq_vector_pi/2(uq_ctrl) -> dq2alphabeta/2(q)
